simulink model "Speed_Torque_Trace_Generator"  (R2016b)
settings: Solver=FixedStepDiscrete  StartTime=0.0  StopTime=inf  FixedStep=SpdTqTrcGenr.tiSimnTiStep_C  RelTol=1e-3  EnableMultiTasking=on
settings Model: Creator=m01wolf  LastModifiedBy=sevren
settings DataIOCC: SaveFormat=StructureWithTime  SaveOutput=off  DSMLogging=off  VisualizeSimOutput=off  SaveTime=off  StateSaveName=Results  SignalLoggingName=Results
settings OptimizationCC: BlockReduction=off  ConditionallyExecuteInputs=off  LifeSpan=inf
settings DebuggingCC: AllowSymbolicDim=off  SFUnexpectedBacktrackingDiag=warning  SFNoUnconditionalDefaultTransitionDiag=warning  SFExecutionAtInitializationDiag=none
settings ModelReferenceCC: ModelReferenceNumInstancesAllowed=Single  PropagateSignalLabelsOutOfModel=off
settings GRTTargetCC: TargetLangStandard=C89/C90 (ANSI)
settings ConfigComp: CovMetricSettings=dw  CovHtmlReporting=on  CovSaveCumulativeToWorkspaceVar=on  CovSaveSingleToWorkspaceVar=on  CovExternalEMLEnable=off

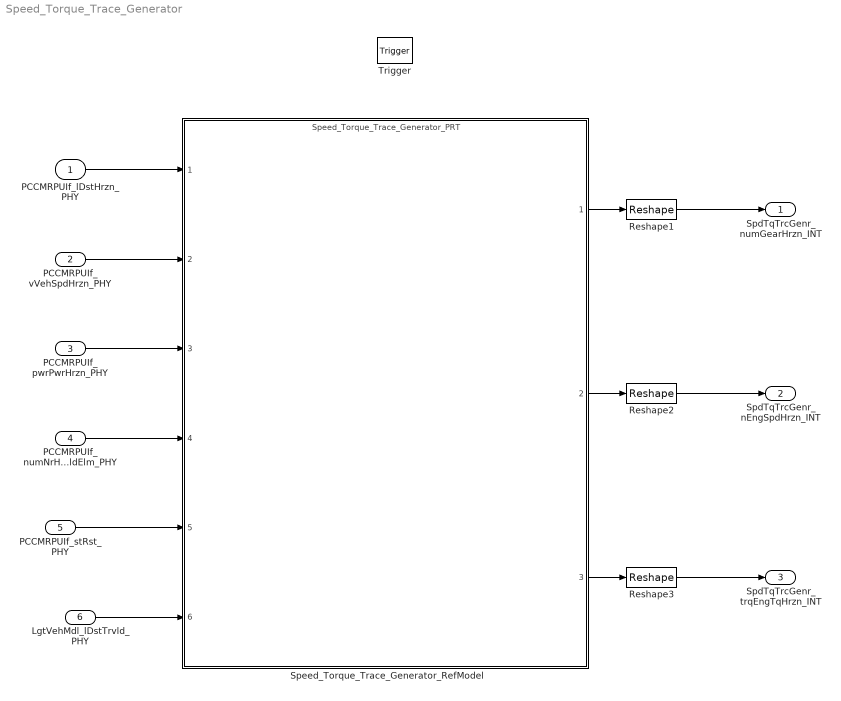
== system Speed_Torque_Trace_Generator ==
  PCCMRPUIf_lDstHrzn_PHY : Inport
  PCCMRPUIf_vVehSpdHrzn_PHY : Inport  Port=2
  PCCMRPUIf_pwrPwrHrzn_PHY : Inport  Port=3
  PCCMRPUIf_numNrHrznVldElm_PHY : Inport  Port=4
  PCCMRPUIf_stRst_PHY : Inport  Port=5
  LgtVehMdl_lDstTrvld_PHY : Inport  Port=6
  Trigger : TriggerPort  TriggerType=function-call  VariantControl=Variant  PortDimensions=1
  Reshape1 : Reshape  OutputDimensionality=Column vector (2-D)
  Reshape2 : Reshape  OutputDimensionality=Column vector (2-D)
  Reshape3 : Reshape  OutputDimensionality=Column vector (2-D)
  Speed_Torque_Trace_Generator_RefModel : ModelReference  ModelNameDialog=Speed_Torque_Trace_Generator_PRT.slxp  ModelReferenceVersion=1.271  CopyOfModelProtected=on
  SpdTqTrcGenr_numGearHrzn_INT : Outport  PortDimensions=[400,1]
  SpdTqTrcGenr_nEngSpdHrzn_INT : Outport  Port=2  PortDimensions=[400,1]
  SpdTqTrcGenr_trqEngTqHrzn_INT : Outport  Port=3  PortDimensions=[400,1]
  wires:
  Speed_Torque_Trace_Generator_RefModel/1 -> Reshape1/1
  Speed_Torque_Trace_Generator_RefModel/2 -> Reshape2/1
  Speed_Torque_Trace_Generator_RefModel/3 -> Reshape3/1
  PCCMRPUIf_lDstHrzn_PHY/1 -> Speed_Torque_Trace_Generator_RefModel/1
  PCCMRPUIf_vVehSpdHrzn_PHY/1 -> Speed_Torque_Trace_Generator_RefModel/2
  PCCMRPUIf_pwrPwrHrzn_PHY/1 -> Speed_Torque_Trace_Generator_RefModel/3
  PCCMRPUIf_numNrHrznVldElm_PHY/1 -> Speed_Torque_Trace_Generator_RefModel/4
  PCCMRPUIf_stRst_PHY/1 -> Speed_Torque_Trace_Generator_RefModel/5
  Reshape1/1 -> SpdTqTrcGenr_numGearHrzn_INT/1
  Reshape2/1 -> SpdTqTrcGenr_nEngSpdHrzn_INT/1
  Reshape3/1 -> SpdTqTrcGenr_trqEngTqHrzn_INT/1
  LgtVehMdl_lDstTrvld_PHY/1 -> Speed_Torque_Trace_Generator_RefModel/6
